simulink model "gas_pipeline_vs2_secure"  (Simulink 9.2)
settings: Solver=ode45  StartTime=0.0  StopTime=10  RelTol=1e-3  EnableMultiTasking=on
undefined symbols (not defined in the file): Tab, Tba, Tca, Tcb
settings Model: Creator=Luan Nguyen  LastModifiedBy=gautam
settings OptimizationCC: ExpressionDepthLimit=2147483647
settings DebuggingCC: IgnoredZcDiagnostic=none  MultiTaskDSMMsg=warning  MultiTaskCondExecSysMsg=none  FcnCallInpInsideContextMsg=error
settings GRTTargetCC: CombineOutputUpdateFcns=on  GRTInterface=off
settings ConfigComp: CovSFcnEnable=off

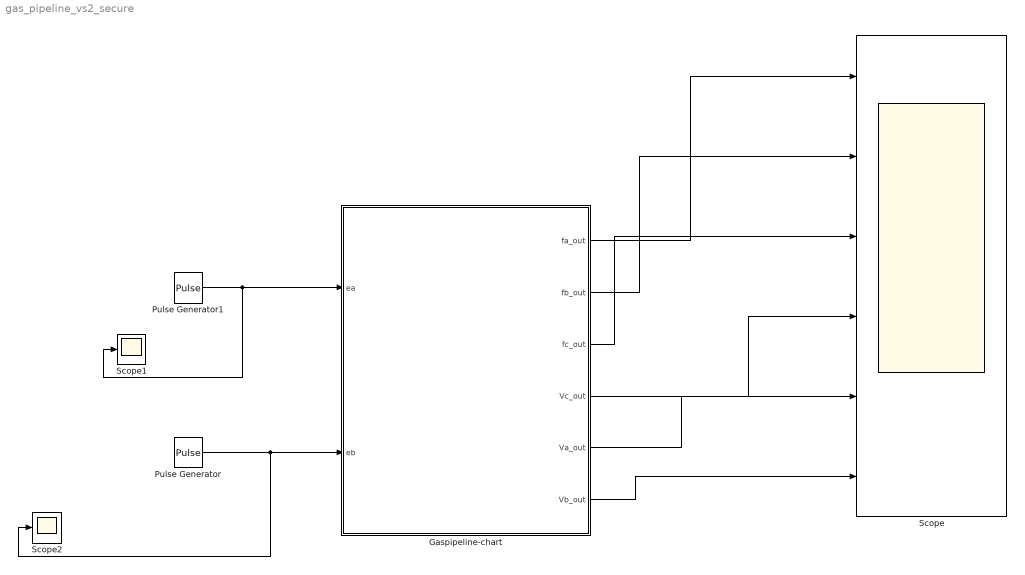
== system gas_pipeline_vs2_secure ==
  Gaspipeline-chart : Stateflow chart  TreatAsAtomicUnit=on
  Pulse Generator : DiscretePulseGenerator  PulseType=Time based  Amplitude=3  Period=10
  Pulse Generator1 : DiscretePulseGenerator  PulseType=Time based  Amplitude=-3  Period=10
  Scope : Scope  NumInputPorts=6
  Scope1 : Scope
  Scope2 : Scope
  wires:
  Gaspipeline-chart/1(fa_out) -> Scope/1
  Gaspipeline-chart/2(fb_out) -> Scope/2
  Gaspipeline-chart/3(fc_out) -> Scope/3
  Gaspipeline-chart/4(Vc_out) -> Scope/4
  Gaspipeline-chart/5(Va_out) -> Scope/5
  Gaspipeline-chart/6(Vb_out) -> Scope/6
  Pulse Generator1/1 -> Scope1/1, Gaspipeline-chart/1(ea)
  Pulse Generator/1 -> Scope2/1, Gaspipeline-chart/2(eb)

== stateflow chart Gaspipeline-chart ==
  settings: updateMethod=CONTINUOUS
  state B_controller [parallel]
    settings: executionOrder=1
    state ModeB1
      du:
      zb_dot = 1;
    state ModeB3
      du:
      zb_dot = 1;
    state ModeB2
      du:
      zb_dot = 1;
    (default) -> ModeB1 : {fb = 5; fc = 10; fa = 5; zb = 0; tmpB = 0;}
    ModeB1 -> ModeB2 [order 1] : [eb >= 0]{tmpB = eb;zb = 0;}
    ModeB3 -> ModeB1 : [zb >= 1]
        | {fb = fb+ tmpB;zb = 0;}
    ModeB2 -> ModeB1 : [zb >= Tcb]
        | {fb = fb+tmpB; zb = 0;}
    ModeB1 -> ModeB3 [order 2] : [eb <= 0 ]
        | {tmpB = eb;zb = 0;}
  state A_controller [parallel]
    settings: executionOrder=2
    state ModeA5
      du:
      za_dot = 1;
    state ModeA2
      du:
      za_dot = 1;
    state ModeA1
      du:
      za_dot = 1;
    (default) -> ModeA1 : {za = 0;tmpA = 0;}
    ModeA1 -> ModeA2 [order 1] : [ea > 0]{tmpA = ea;za = 0;}
    ModeA5 -> ModeA1 : [za >= 1]
        | {fa = fa+ tmpA;za = 0;}
    ModeA2 -> ModeA1 : [za >= Tca]
        | {fa = fa+tmpA; za = 0;}
    ModeA1 -> ModeA5 [order 2] : [ea <= 0 ]
        | {tmpA = ea;za = 0}
  state C_controller [parallel]
    settings: executionOrder=3
    state C2
      du:
      zc_dot = 1;
    state C1
      du:
      zc_dot = 1;
    (default) -> C1 : {zc = 0; tmpC = 0;}
    C2 -> C1 : [zc >=1]
        | {fc = fc+tmpC; zc = 0;}
    C1 -> C2 : [ea +eb >0 || ea + eb <0]
        | {tmpC = ea+eb;}
  state PlantModel [parallel]
    settings: executionOrder=4
    state Plant
      du:
      Va_dot = fa; Va_out = Va; fa_dot = 0; fa_out = fa;
      Vb_dot = fb; Vb_out = Vb; fb_dot = 0; fb_out = fb;
      Vc_dot = fc; Vc_out = Vc; fc_dot = 0; fc_out = fc;
  data: za local double; zb local double; fa local double; fa_out output double; ea input double; fb local double; fb_out output double; fc local double; fc_out output double; Va local double; Vb local double; Vc local double; Vc_out output double; Va_out output double; Vb_out output double; Tba parameter double; Tca parameter double; Tcb parameter double; eb input double; Tab parameter double; zc local double; tmpA local double; tmpB local double; tmpC local double
  data za settings: updateMethod=SF_CONTINUOUS_TIME_DATA
  data zb settings: updateMethod=SF_CONTINUOUS_TIME_DATA
  data fa settings: updateMethod=SF_CONTINUOUS_TIME_DATA
  data fb settings: updateMethod=SF_CONTINUOUS_TIME_DATA
  data fc settings: updateMethod=SF_CONTINUOUS_TIME_DATA
  data Va settings: updateMethod=SF_CONTINUOUS_TIME_DATA
  data Vb settings: updateMethod=SF_CONTINUOUS_TIME_DATA
  data Vc settings: updateMethod=SF_CONTINUOUS_TIME_DATA
  data zc settings: updateMethod=SF_CONTINUOUS_TIME_DATA
